simulink model "Reconstruction_model"  (R2021a)
settings: Solver=VariableStepAuto  StartTime=0.0  StopTime=10.0  RelTol=1e-3
values from neighbouring files (symbols this model uses):
  xp = x    [L1_4_sec_fft.m]    (also in L1_5_sec_dst.m; L1_5sec_dct.m; L1_dct_6_sec.m; L1_dst_4_sec.m)
settings Model: Creator=yadu1  LastModifiedBy=sumuk

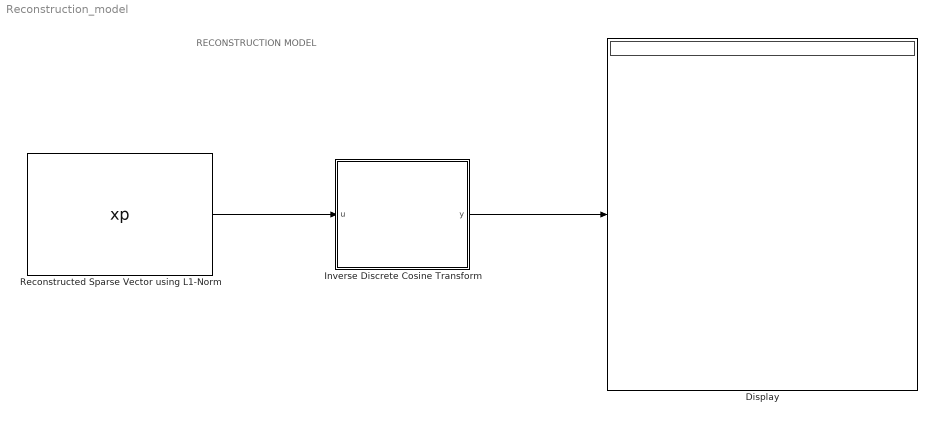
== system Reconstruction_model ==
  note: RECONSTRUCTION MODEL
  Display : Display
  Inverse Discrete Cosine Transform : MATLAB Function  TreatAsAtomicUnit=on
  Reconstructed Sparse Vector using L1-Norm : Constant  Value=xp
  wires:
  Inverse Discrete Cosine Transform/1(y) -> Display/1
  Reconstructed Sparse Vector using L1-Norm/1 -> Inverse Discrete Cosine Transform/1(u)

== matlab function Reconstruction_model/Inverse Discrete Cosine Transform ==
  data: u input; y output
function y = idct(u)

y = u;
